simulink model "sys2nd"  (R2015b)
settings: Solver=VariableStepAuto  StartTime=0.0  StopTime=5  RelTol=1e-3
settings Model: Creator=Xiong  LastModifiedBy=Xiong

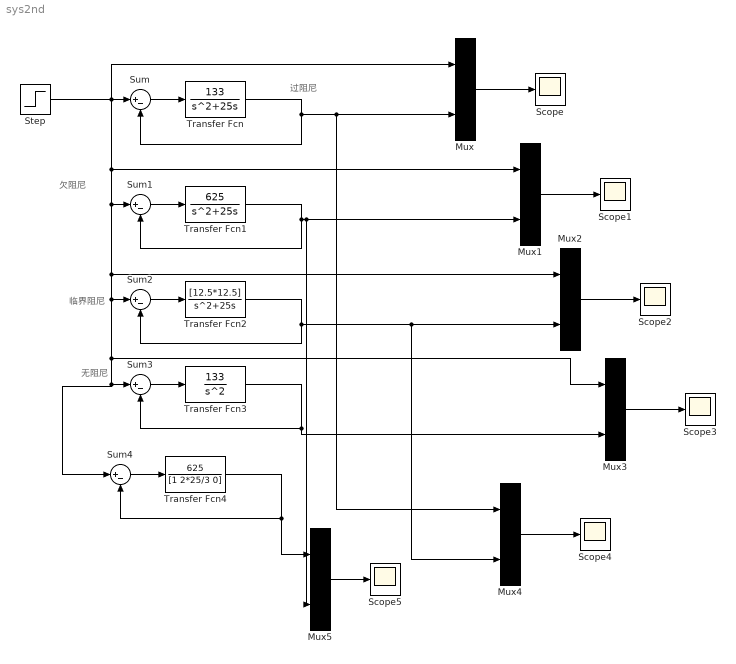
== system sys2nd ==
  note: 无阻尼
  note: 临界阻尼
  note: 过阻尼
  note: 欠阻尼
  Mux{,1..5} (6 alike) : Mux  Inputs=2
  Scope{,1..5} (6 alike) : Scope
  Step : Step  SampleTime=0
  Sum{,1..4} (5 alike) : Sum  Inputs=|+-
  Transfer Fcn : TransferFcn  Numerator=[133]  Denominator=[1 25 0]
  Transfer Fcn1 : TransferFcn  Numerator=[625]  Denominator=[1 25 0]
  Transfer Fcn2 : TransferFcn  Numerator=[12.5*12.5]  Denominator=[1 25 0]
  Transfer Fcn3 : TransferFcn  Numerator=[133]  Denominator=[1 0 0]
  Transfer Fcn4 : TransferFcn  Numerator=[625]  Denominator=[1 2*25/3 0]
  wires:
  Mux/1 -> Scope/1
  Sum/1 -> Transfer Fcn/1
  Transfer Fcn1/1 -> Mux1/2, Mux5/2, Sum1/2
  Sum1/1 -> Transfer Fcn1/1
  Sum2/1 -> Transfer Fcn2/1
  Transfer Fcn3/1 -> Mux3/2, Sum3/2
  Sum3/1 -> Transfer Fcn3/1
  Mux1/1 -> Scope1/1
  Mux2/1 -> Scope2/1
  Mux3/1 -> Scope3/1
  Transfer Fcn2/1 -> Mux4/2, Mux2/2, Sum2/2
  Transfer Fcn/1 -> Mux4/1, Mux/2, Sum/2
  Mux4/1 -> Scope4/1
  Transfer Fcn4/1 -> Mux5/1, Sum4/2
  Sum4/1 -> Transfer Fcn4/1
  Step/1 -> Mux1/1, Mux2/1, Sum4/1, Sum3/1, Mux3/1, Sum2/1, Sum1/1, Mux/1, Sum/1
  Mux5/1 -> Scope5/1
